simulink model "annotations"  (Simulink 7.8)
settings: Solver=ode45  SolverMode=SingleTasking  StartTime=0.0  StopTime=10.0  RelTol=1e-3
libraries: simulink x1
settings Model: Creator=GM  LastModifiedBy=GM  CovMetricSettings=dwe  CovHtmlReporting=off  covSaveCumulativeToWorkspaceVar=off  CovSaveSingleToWorkspaceVar=off  CovExternalEMLEnable=on
settings DataIOCC: LimitDataPoints=off  SaveFormat=StructureWithTime  SignalLoggingSaveFormat=Dataset
settings OptimizationCC: ExpressionDepthLimit=128
settings DebuggingCC: UnderspecifiedInitializationDetection=Simplified  MergeDetectMultiDrivingBlocksExec=error  SolverPrmCheckMsg=none  FrameProcessingCompatibilityMsg=error  StateNameClashWarn=none  SFUnexpectedBacktrackingDiag=error  SFNoUnconditionalDefaultTransitionDiag=error
settings HardwareCC: ProdBitPerPointer=64  ProdLargestAtomicFloat=Float  ProdIntDivRoundTo=Zero  ProdEndianess=LittleEndian  ProdHWDeviceType=Specified
settings CodeAppCC: CustomSymbolStrType=$N$R$M_T
settings GRTTargetCC: TargetFunctionLibrary=C99 (ISO)  GeneratePreprocessorConditionals=Use local settings

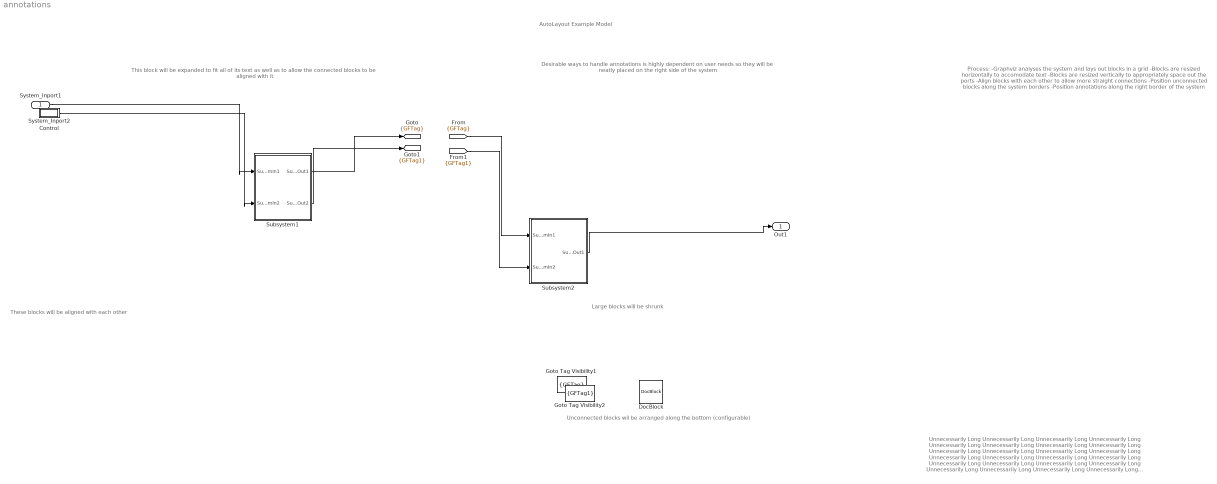
== system annotations ==
  note: Process:
      | -Graphviz analyses the system and lays out blocks in a grid
      |
      | -Blocks are resized horizontally to accomodate text
      |
      | -Blocks are resized vertically to appropriately space out the ports
      |
      | -Align blocks with each other to allow more straight connections
      |
      | -Position unconnected blocks along the system borders
      |
      | -Position annotations along the right border of the system
  note: These blocks will be aligned with each other
  note: Desirable ways to handle annotations is highly dependent on user needs
      | so they will be neatly placed on the right side of the system
  note: This block will be expanded to fit all of its text
      | as well as to allow the connected blocks to be aligned with it
  note: Large blocks will be shrunk
  note: AutoLayout Example Model
  note: Unconnected blocks wil be arranged along the bottom (configurable)
  note: Unnecessarily Long Unnecessarily Long Unnecessarily Long Unnecessarily Long
      |
      | Unnecessarily Long Unnecessarily Long Unnecessarily Long Unnecessarily Long
      |
      | Unnecessarily Long Unnecessarily Long Unnecessarily Long Unnecessarily Long
      |
      | Unnecessarily Long Unnecessarily Long Unnecessarily Long Unnecessarily Long
      |
      | Unnecessarily Long Unnecessarily Long Unnecessarily Long Unnecessarily Long
      |
      | Unnecessarily Long Unnecessarily Long Unnecessarily Long Unnecessarily Long
      |
      | Unnecessarily Long Unnecessarily Long Unnecessarily Long Unnecessarily Long
      |
      | Unnecessarily Long Unnecessarily Long Unnecessarily Long Unnecessarily Long
      |
      | Unnecessarily Long Unnecessarily Long Unnecessarily Long Unnecessarily Long
      |
      | Unnecessarily Long Unnecessarily Long Unnecessarily Long Unnecessarily Long
      |
      | Unnecessarily Long Unnecessarily Long Unnecessarily Long Unnecessarily Long
      |
      | Unnecessarily Long Unnecessarily Long Unnecessarily Long Unnecessarily Long
      |
      | Unnecessarily Long Unnecessarily Long Unnecessarily Long Unnecessarily Long
      |
      | Unnecessarily Long Unnecessarily Long Unnecessarily Long Unnecessarily Long
      |
      | Unnecessarily Long Unnecessarily Long Unnecessarily Long Unnecessarily Long
      |
      | Unnecessarily Long Unnecessarily Long Unnecessarily Long Unnecessarily Long
      |
      | Unnecessarily Long Unnecessarily Long Unnecessarily Long Unnecessarily Long
      |
      | Unnecessarily Long Unnecessarily Long Unnecessarily Long Unnecessarily Long
      |
      | Unnecessarily Long Unnecessarily Long Unnecessarily Long Unnecessarily Long
      |
      | Unnecessarily Long Unnecessarily Long Unnecessarily Long Unnecessarily Long
      |
      | Unnecessarily Long Unnecessarily Long Unnecessarily Long Unnecessarily Long
      |
      | Unnecessarily Long Unnecessarily Long Unnecessarily Long Unnecessarily Long
      |
      | Unnecessarily Long Unnecessarily Long Unnecessarily Long Unnecessarily Long
      |
      | Unnecessarily Long Unnecessarily Long Unnecessarily Long Unnecessarily Long
      |
      | Unnecessarily Long Unnecessarily Long Unnecessarily Long Unnecessarily Long
      |
      | Unnecessarily Long Unnecessarily Long Unnecessarily Long Unnecessarily Long
      |
      | Unnecessarily Long Unnecessarily Long Unnecessarily Long Unnecessarily Long
      |
      | Unnecessarily Long Unnecessarily Long Unnecessarily Long Unnecessarily Long
      |
      | Unnecessarily Long Unnecessarily Long Unnecessarily Long Unnecessarily Long
      |
      | Unnecessarily Long Unnecessarily Long Unnecessarily Long Unnecessarily Long
      |
      | Unnecessarily Long Unnecessarily Long Unnecessarily Long Unnecessarily Long
      |
      | Unnecessarily Long Unnecessarily Long Unnecessarily Long Unnecessarily Long
      |
      | Unnecessarily Long Unnecessarily Long Unnecessarily Long Unnecessarily Long
      |
      | Unnecessarily Long Unnecessarily Long Unnecessarily Long Unnecessarily Long
      |
      | Unnecessarily Long Unnecessarily Long Unnecessarily Long Unnecessarily Long
      |
      | Unnecessarily Long Unnecessarily Long Unnecessarily Long Unnecessarily Long
      |
      | Unnecessarily Long Unnecessarily Long Unnecessarily Long Unnecessarily Long
  System_Inport1 : Inport  OutDataTypeStr=single
  System_Inport2 : Inport  Port=2  OutDataTypeStr=single
  Control : Subsystem  AncestorBlock=ESSR/ESSR/Control
  DocBlock : simulink/Model-Wide Utilities/DocBlock  ECoderFlag=DocBlock  DocumentType=RTF
  Goto Tag Visibility1 : GotoTagVisibility  GotoTag=GFTag
  Goto Tag Visibility2 : GotoTagVisibility  GotoTag=GFTag1
  Subsystem1 : Subsystem  AncestorBlock=ESSR/ESSR/ESSI
  Subsystem2 : Subsystem  AncestorBlock=ESSR/ESSR/ESSI
  Out1 : Outport
  tag scope: GFTag1=scoped, GFTag=scoped
  wires:
  Subsystem2/1(SubsystemOut1) -> Out1/1
  [GFTag1] -> Subsystem2/2(SubsystemIn2)
  [GFTag] -> Subsystem2/1(SubsystemIn1)
  System_Inport2/1 -> Subsystem1/2(SubsystemIn2)
  System_Inport1/1 -> Subsystem1/1(SubsystemIn1)
  Subsystem1/1(SubsystemOut1) -> [GFTag]
  Subsystem1/2(SubsystemOut2) -> [GFTag1]

== system annotations/Control ==

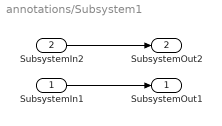
== system annotations/Subsystem1 ==
  SubsystemIn1 : Inport
  SubsystemIn2 : Inport  Port=2
  SubsystemOut1 : Outport
  SubsystemOut2 : Outport  Port=2
  wires:
  SubsystemIn1/1 -> SubsystemOut1/1
  SubsystemIn2/1 -> SubsystemOut2/1

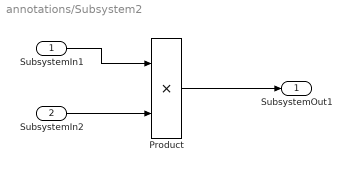
== system annotations/Subsystem2 ==
  SubsystemIn1 : Inport
  SubsystemIn2 : Inport  Port=2
  Product : Product
  SubsystemOut1 : Outport
  wires:
  SubsystemIn1/1 -> Product/1
  SubsystemIn2/1 -> Product/2
  Product/1 -> SubsystemOut1/1
